simulink subsystem "vessel_compliance"  (R2020b)
settings: Solver=VariableStepAuto  StartTime=0.0  StopTime=10.0  RelTol=1e-3
settings Model: Creator=RH  LastModifiedBy=Marco

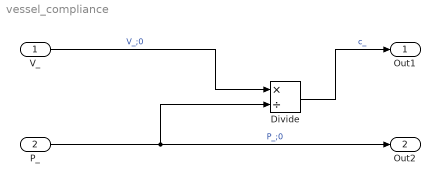
== system vessel_compliance ==
  V_ : Inport  Unit=L
  P_ : Inport  Port=2  Unit=mmHg
  Divide : Product  Inputs=*/
  Out1 : Outport  Unit=L/mmHg
  Out2 : Outport  Port=2  Unit=mmHg
  wires:
  Divide/1 -> Out1/1  "c_"
  P_/1 -> Out2/1, Divide/2  "P_;0"
  V_/1 -> Divide/1  "V_;0"
